simulink model "image_analysis_hough"  (Simulink 7.6)
settings: Solver=FixedStepDiscrete  StartTime=0.0  StopTime=0  RelTol=1e-3
undefined symbols (not defined in the file or in its folder): jet, Rec, SDTV
libraries: vipsnks x2, vipconversions x1, vipsrcs x1
settings Model: Creator=Administrator  LastModifiedBy=Administrator

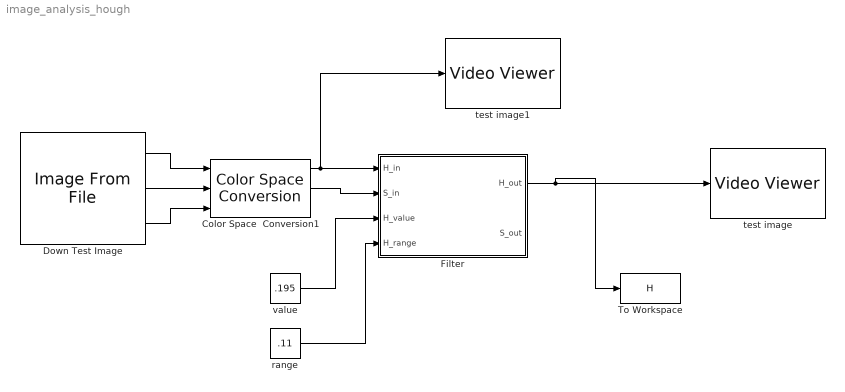
== system image_analysis_hough ==
  Color Space  Conversion1 : vipconversions/Color Space  Conversion  conversion=Obsolete  conversionActive=R'G'B' to HSV  wp_str=D65  rec=Rec. 601 (SDTV)  sys=1125/60/2:1  imagePorts=Separate color signals
  Down Test Image : vipsrcs/Image From File  Tag=vipblks_nd  DialogController=vipDDGCreate  DialogControllerArgs=DataTag0  SystemSampleTime=-1  FileName=C:\Documents and Settings\Administrator\My Documents\Academics\Summer 2011\AUVT\Pool Tests\6-1-11\image7.PNG  imagePorts=Separate color signals  Ts=-1  ImageDataType=double  Signed=on  WordLength=16  sdImageDataType=uint(8)  FractionLengthMode=User-defined  FractionLength=15  OutPortLabels=R|G|B
  Filter : Stateflow chart  TreatAsAtomicUnit=on
  To Workspace : ToWorkspace  VariableName=H  SampleTime=-1  SaveFormat=Array
  range : Constant  Value=.11  SampleTime=-1
  test image : vipsnks/Video Viewer  DialogControllerArgs=DataTag2  inputType=Obsolete7b  imagePorts=One multidimensional signal  useColorMap=off  colormapValue=jet(256)  specRange=off  minInputVal=0  maxInputVal=255  FigPos=[974 421 253 210]  AxisZoom=on  trueSizedOnce=off  OpenAtMdlStart=on
  test image1 : vipsnks/Video Viewer  DialogControllerArgs=DataTag4  inputType=Obsolete7b  imagePorts=One multidimensional signal  useColorMap=off  colormapValue=jet(256)  specRange=off  minInputVal=0  maxInputVal=255  FigPos=[864 420 269 154]  AxisZoom=on  trueSizedOnce=off  OpenAtMdlStart=on
  value : Constant  Value=.195  SampleTime=-1
  wires:
  Down Test Image/1 -> Color Space  Conversion1/1
  Down Test Image/2 -> Color Space  Conversion1/2
  Down Test Image/3 -> Color Space  Conversion1/3
  Color Space  Conversion1/1 -> Filter/1(H_in), test image1/1
  Color Space  Conversion1/2 -> Filter/2(S_in)
  Filter/1(H_out) -> test image/1, To Workspace/1
  value/1 -> Filter/3(H_value)
  range/1 -> Filter/4(H_range)

== matlab function Filter ==
  data: H_in input double; S_in input double; H_value input double; H_range input double; H_out output double; S_out output double
function [H_out, S_out] = path_filter(H_in, S_in, H_value, H_range)  %H_lower, H_upper)
% This function extracts the pixels containing hues that path elements are
%   expected to have


% Initialize
H_out = double(H_in);
S_out = double(S_in);

H_lower = H_value - H_range/2;
H_upper = H_value + H_range/2;


% Set values outside valid ranges to zero
for i = 1:size(H_in,1)
    for j = 1:size(H_in,2)
        
        if( H_in(i,j) >= H_lower && H_in(i,j) <= H_upper )
            H_out(i,j) = 1;
        else
            H_out(i,j) = 0;
        end
        
    end
end



return
